simulink model "ADA"  (R2019b)
settings: Solver=FixedStepAuto  StartTime=0.0  StopTime=10.0  FixedStep=fixedStepSize  RelTol=1e-3
undefined symbols (not defined in the file): ADA_notAlwaysHorizon, ADA_subsystem1_rpmLimit, ADA_subsystem1_timeHorizon, ADA_subsystem2_gear1, ADA_subsystem2_gear2, ADA_subsystem2_impellerMax, ADA_subsystem2_impellerMin, ADA_subsystem2_maxValue, ADA_subsystem2_throttleMin, ADA_subsystem3_gear, ADA_subsystem3_gearSelectionState, ADA_subsystem3_speedMax, ADA_subsystem3_speedMin, fixedStepSize
libraries: simulink x1
settings Model: Creator=JEDDELAN  LastModifiedBy=alex
settings DataIOCC: SaveOutput=off  SaveTime=off  ReturnWorkspaceOutputs=off
settings DebuggingCC: ArithmeticOperatorsInVariantConditions=warning
settings SFSimCC: SimUseLocalCustomCode=off  CustomCodeUndefinedFunction=UseInterfaceOnly
settings RTWCC: RTWUseLocalCustomCode=off
settings GRTTargetCC: CombineOutputUpdateFcns=off  MatFileLogging=off

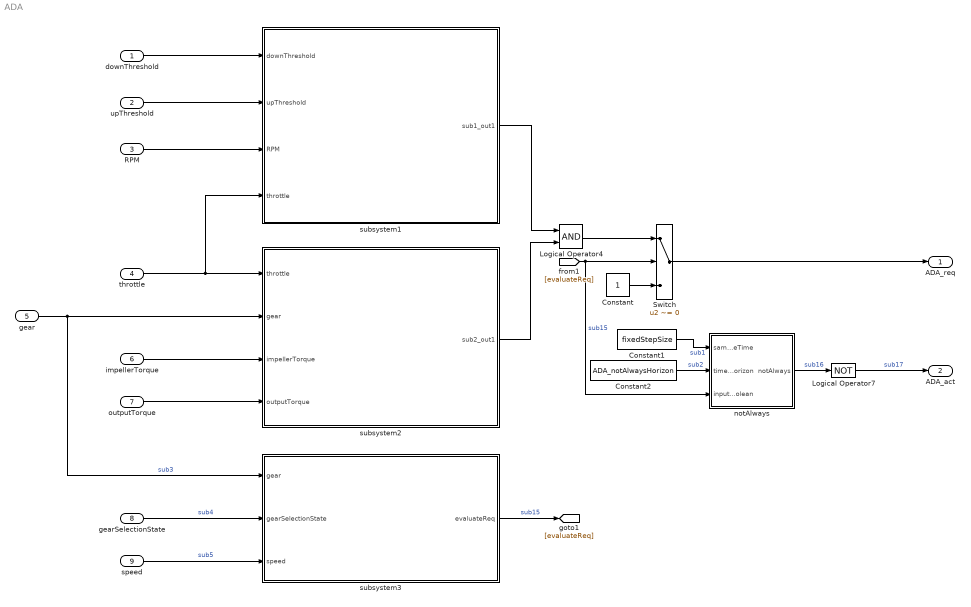
== system ADA ==
  downThreshold : Inport  OutDataTypeStr=double
  upThreshold : Inport  Port=2  OutDataTypeStr=double
  RPM : Inport  Description=|  Port=3  OutDataTypeStr=double  PortDimensions=1  BusOutputAsStruct=on
      | Engine Speed [rpm]
      | Engine Speed derivative [rpm/s]
  throttle : Inport  Port=4
  gear : Inport  Port=5
  impellerTorque : Inport  Port=6
  outputTorque : Inport  Port=7
  gearSelectionState : Inport  Port=8
  speed : Inport  Port=9
  Constant : Constant  OutDataTypeStr=boolean
  Constant1 : Constant  Value=fixedStepSize
  Constant2 : Constant  Value=ADA_notAlwaysHorizon
  Logical Operator4 : Logic  AllPortsSameDT=off  OutDataTypeStr=boolean
  Logical Operator7 : Logic  Operator=NOT  AllPortsSameDT=off  OutDataTypeStr=boolean
  Switch : Switch  Criteria=u2 ~= 0
  notAlways : Subsystem
      settings: CopyFcn=set_param(gcbh,'LinkStatus','none');
  subsystem1 : Subsystem
  subsystem2 : Subsystem
  subsystem3 : Subsystem
  ADA_req : Outport  OutDataTypeStr=boolean  PortDimensions=1  VectorParamsAs1DForOutWhenUnconnected=off
  ADA_act : Outport  Port=2  OutDataTypeStr=boolean  PortDimensions=1  VectorParamsAs1DForOutWhenUnconnected=off
  wires:
  notAlways/1(notAlways) -> Logical Operator7/1  "sub16"
  [evaluateReq] -> Switch/2, notAlways/3(inputBoolean)  "sub15"
  Logical Operator4/1 -> Switch/1
  speed/1 -> subsystem3/3(speed)  "sub5"
  upThreshold/1 -> subsystem1/2(upThreshold)
  Logical Operator7/1 -> ADA_act/1  "sub17"
  throttle/1 -> subsystem2/1(throttle), subsystem1/4(throttle)
  impellerTorque/1 -> subsystem2/3(impellerTorque)
  RPM/1 -> subsystem1/3(RPM)
  subsystem3/1(evaluateReq) -> [evaluateReq]  "sub15"
  outputTorque/1 -> subsystem2/4(outputTorque)
  gear/1 -> subsystem3/1(gear), subsystem2/2(gear)  "sub3"
  Constant1/1 -> notAlways/1(sampleTime)  "sub1"
  subsystem2/1(sub2_out1) -> Logical Operator4/2
  Constant/1 -> Switch/3
  Switch/1 -> ADA_req/1
  gearSelectionState/1 -> subsystem3/2(gearSelectionState)  "sub4"
  Constant2/1 -> notAlways/2(timeHorizon)  "sub2"
  downThreshold/1 -> subsystem1/1(downThreshold)
  subsystem1/1(sub1_out1) -> Logical Operator4/1

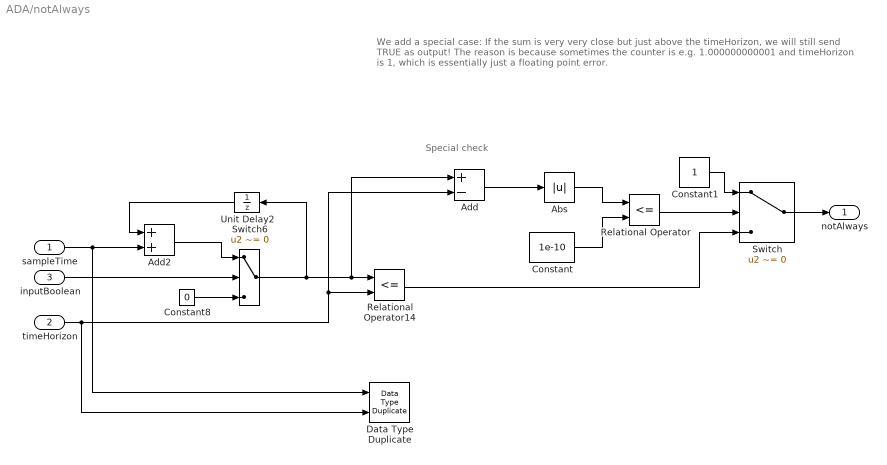
== system ADA/notAlways ==
  note: Special check
  note: We add a special case:
      | If the sum is very very close but just above the timeHorizon, we will still send TRUE as output!
      |
      | The reason is because sometimes the counter is e.g. 1.000000000001 and timeHorizon is 1, which is essentially just a floating point error.
  sampleTime : Inport
  timeHorizon : Inport  Port=2
  inputBoolean : Inport  Port=3
  Abs : Abs
  Add : Sum  Inputs=+-
  Add2 : Sum
  Constant : Constant  Value=1e-10
  Constant1 : Constant  OutDataTypeStr=boolean
  Constant8 : Constant  Value=0  OutDataTypeStr=Inherit: Inherit via back propagation
  Data Type Duplicate : DataTypeDuplicate
  Relational Operator : RelationalOperator  Operator=<=  OutDataTypeStr=boolean  RndMeth=Simplest
  Relational Operator14 : RelationalOperator  Operator=<=  OutDataTypeStr=boolean  RndMeth=Nearest
  Switch : Switch  Criteria=u2 ~= 0
  Switch6 : Switch  Criteria=u2 ~= 0
  Unit Delay2 : UnitDelay  SampleTime=-1  HasFrameUpgradeWarning=on
  notAlways : Outport  VectorParamsAs1DForOutWhenUnconnected=off
  wires:
  Switch6/1 -> Add/1, Relational Operator14/1, Unit Delay2/1
  timeHorizon/1 -> Add/2, Relational Operator14/2, Data Type Duplicate/2
  Relational Operator14/1 -> Switch/3
  Unit Delay2/1 -> Add2/1
  Add2/1 -> Switch6/1
  sampleTime/1 -> Add2/2, Data Type Duplicate/1
  Constant8/1 -> Switch6/3
  inputBoolean/1 -> Switch6/2
  Add/1 -> Abs/1
  Abs/1 -> Relational Operator/1
  Constant/1 -> Relational Operator/2
  Relational Operator/1 -> Switch/2
  Constant1/1 -> Switch/1
  Switch/1 -> notAlways/1

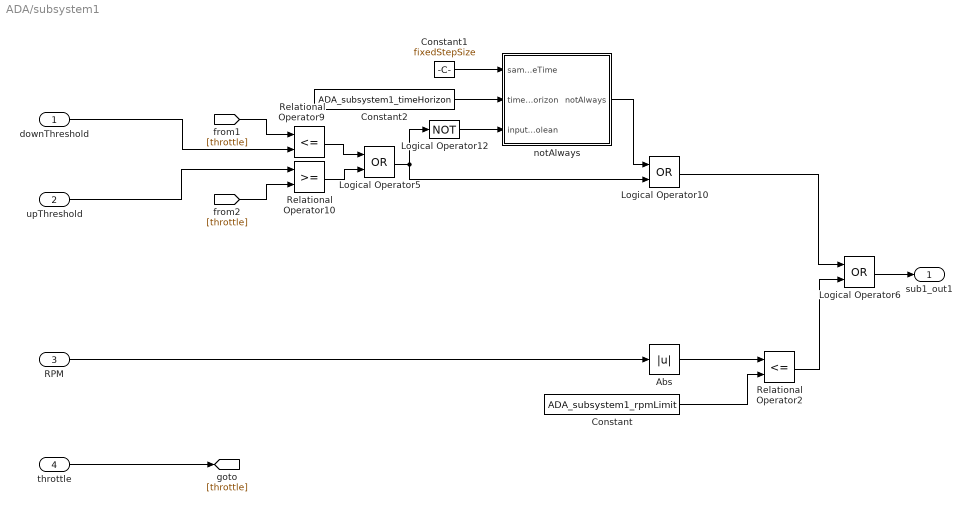
== system ADA/subsystem1 ==
  downThreshold : Inport
  upThreshold : Inport  Port=2
  RPM : Inport  Port=3
  throttle : Inport  Port=4
  Abs : Abs
  Constant : Constant  Value=ADA_subsystem1_rpmLimit
  Constant1 : Constant  Value=fixedStepSize
  Constant2 : Constant  Value=ADA_subsystem1_timeHorizon
  Logical Operator10 : Logic  Operator=OR  AllPortsSameDT=off  OutDataTypeStr=boolean
  Logical Operator12 : Logic  Operator=NOT  AllPortsSameDT=off  OutDataTypeStr=boolean
  Logical Operator5 : Logic  Operator=OR  AllPortsSameDT=off  OutDataTypeStr=boolean
  Logical Operator6 : Logic  Operator=OR  AllPortsSameDT=off  OutDataTypeStr=boolean
  Relational Operator10 : RelationalOperator  OutDataTypeStr=boolean  RndMeth=Nearest
  Relational Operator2 : RelationalOperator  Operator=<=  OutDataTypeStr=boolean  RndMeth=Nearest
  Relational Operator9 : RelationalOperator  Operator=<=  OutDataTypeStr=boolean  RndMeth=Nearest
  notAlways : Subsystem
      settings: CopyFcn=set_param(gcbh,'LinkStatus','none');
  sub1_out1 : Outport  VectorParamsAs1DForOutWhenUnconnected=off
  wires:
  throttle/1 -> [throttle]
  notAlways/1(notAlways) -> Logical Operator10/1
  Constant2/1 -> notAlways/2(timeHorizon)
  Constant1/1 -> notAlways/1(sampleTime)
  Logical Operator12/1 -> notAlways/3(inputBoolean)
  Logical Operator5/1 -> Logical Operator10/2, Logical Operator12/1
  Logical Operator10/1 -> Logical Operator6/1
  RPM/1 -> Abs/1
  Constant/1 -> Relational Operator2/2
  Abs/1 -> Relational Operator2/1
  Relational Operator2/1 -> Logical Operator6/2
  downThreshold/1 -> Relational Operator9/2
  [throttle] -> Relational Operator9/1
  Relational Operator9/1 -> Logical Operator5/1
  [throttle] -> Relational Operator10/2
  Relational Operator10/1 -> Logical Operator5/2
  Logical Operator6/1 -> sub1_out1/1
  upThreshold/1 -> Relational Operator10/1

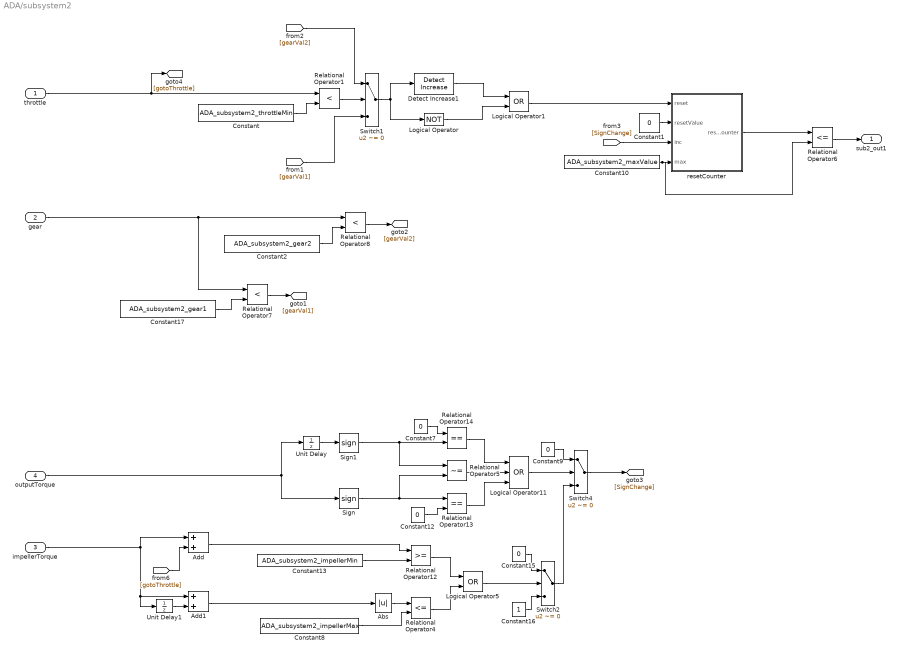
== system ADA/subsystem2 ==
  throttle : Inport
  gear : Inport  Port=2
  impellerTorque : Inport  Port=3
  outputTorque : Inport  Port=4
  Abs : Abs
  Add : Sum
  Add1 : Sum
  Constant : Constant  Value=ADA_subsystem2_throttleMin
  Constant{1,7,9,12,15} (5 alike) : Constant  Value=0
  Constant10 : Constant  Value=ADA_subsystem2_maxValue
  Constant13 : Constant  Value=ADA_subsystem2_impellerMin
  Constant16 : Constant
  Constant17 : Constant  Value=ADA_subsystem2_gear1
  Constant2 : Constant  Value=ADA_subsystem2_gear2
  Constant8 : Constant  Value=ADA_subsystem2_impellerMax
  Detect Increase1 : simulink/Logic and Bit Operations/Detect Increase  vinit=0.0  OutDataTypeStr=boolean
  Logical Operator : Logic  Operator=NOT  AllPortsSameDT=off  OutDataTypeStr=boolean
  Logical Operator1 : Logic  Operator=OR  AllPortsSameDT=off  OutDataTypeStr=boolean
  Logical Operator11 : Logic  Operator=OR  Inputs=3  AllPortsSameDT=off  OutDataTypeStr=boolean
  Logical Operator5 : Logic  Operator=OR  AllPortsSameDT=off  OutDataTypeStr=boolean
  Relational Operator1 : RelationalOperator  Operator=<  OutDataTypeStr=boolean  RndMeth=Nearest
  Relational Operator12 : RelationalOperator  OutDataTypeStr=boolean  RndMeth=Nearest
  Relational Operator13 : RelationalOperator  Operator===  OutDataTypeStr=boolean  RndMeth=Nearest
  Relational Operator14 : RelationalOperator  Operator===  OutDataTypeStr=boolean  RndMeth=Nearest
  Relational Operator4 : RelationalOperator  Operator=<=  OutDataTypeStr=boolean  RndMeth=Nearest
  Relational Operator5 : RelationalOperator  Operator=~=  OutDataTypeStr=boolean  RndMeth=Nearest
  Relational Operator6 : RelationalOperator  Operator=<=  OutDataTypeStr=boolean  RndMeth=Nearest
  Relational Operator7 : RelationalOperator  Operator=<  OutDataTypeStr=boolean  RndMeth=Nearest
  Relational Operator8 : RelationalOperator  Operator=<  OutDataTypeStr=boolean  RndMeth=Nearest
  Sign : Signum
  Sign1 : Signum
  Switch1 : Switch  Criteria=u2 ~= 0
  Switch2 : Switch  Criteria=u2 ~= 0
  Switch4 : Switch  Criteria=u2 ~= 0
  Unit Delay : UnitDelay  SampleTime=-1  HasFrameUpgradeWarning=on
  Unit Delay1 : UnitDelay  SampleTime=-1  HasFrameUpgradeWarning=on
  resetCounter : Subsystem
      settings: CopyFcn=set_param(gcbh,'LinkStatus','none');
  sub2_out1 : Outport  VectorParamsAs1DForOutWhenUnconnected=off
  wires:
  Logical Operator5/1 -> Switch2/2
  Relational Operator4/1 -> Logical Operator5/2
  Abs/1 -> Relational Operator4/1
  Constant8/1 -> Relational Operator4/2
  Add1/1 -> Abs/1
  Unit Delay1/1 -> Add1/2
  Constant7/1 -> Relational Operator14/1
  [SignChange] -> resetCounter/3(inc)
  Logical Operator1/1 -> resetCounter/1(reset)
  throttle/1 -> Relational Operator1/1, [gotoThrottle]
  [gearVal2] -> Switch1/1
  [gearVal1] -> Switch1/3
  Relational Operator1/1 -> Switch1/2
  Constant/1 -> Relational Operator1/2
  Constant15/1 -> Switch2/1
  Switch2/1 -> Switch4/3
  Relational Operator14/1 -> Logical Operator11/1
  Constant12/1 -> Relational Operator13/2
  Relational Operator13/1 -> Logical Operator11/3
  Relational Operator5/1 -> Logical Operator11/2
  Constant16/1 -> Switch2/3
  Logical Operator11/1 -> Switch4/2
  Relational Operator12/1 -> Logical Operator5/1
  Constant13/1 -> Relational Operator12/2
  Add/1 -> Relational Operator12/1
  impellerTorque/1 -> Add/1, Unit Delay1/1, Add1/1
  [gotoThrottle] -> Add/2
  gear/1 -> Relational Operator7/1, Relational Operator8/1
  outputTorque/1 -> Unit Delay/1, Sign/1
  Unit Delay/1 -> Sign1/1
  Sign1/1 -> Relational Operator5/1, Relational Operator14/2
  Sign/1 -> Relational Operator5/2, Relational Operator13/1
  Constant9/1 -> Switch4/1
  Switch4/1 -> [SignChange]
  resetCounter/1(resetCounter) -> Relational Operator6/1
  Constant1/1 -> resetCounter/2(resetValue)
  Constant10/1 -> Relational Operator6/2, resetCounter/4(max)
  Switch1/1 -> Detect Increase1/1, Logical Operator/1
  Detect Increase1/1 -> Logical Operator1/1
  Logical Operator/1 -> Logical Operator1/2
  Relational Operator6/1 -> sub2_out1/1
  Constant17/1 -> Relational Operator7/2
  Constant2/1 -> Relational Operator8/2
  Relational Operator7/1 -> [gearVal1]
  Relational Operator8/1 -> [gearVal2]

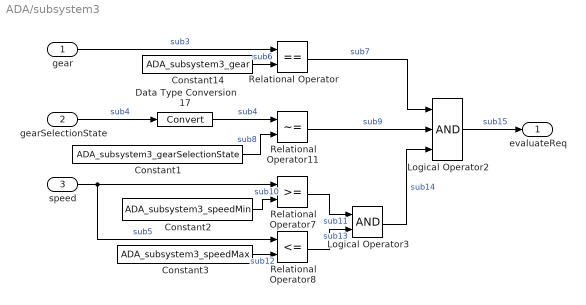
== system ADA/subsystem3 ==
  gear : Inport
  gearSelectionState : Inport  Port=2
  speed : Inport  Port=3
  Constant1 : Constant  Value=ADA_subsystem3_gearSelectionState
  Constant14 : Constant  Value=ADA_subsystem3_gear
  Constant2 : Constant  Value=ADA_subsystem3_speedMin
  Constant3 : Constant  Value=ADA_subsystem3_speedMax
  Data Type Conversion17 : DataTypeConversion
  Logical Operator2 : Logic  Inputs=3  AllPortsSameDT=off  OutDataTypeStr=boolean
  Logical Operator3 : Logic  AllPortsSameDT=off  OutDataTypeStr=boolean
  Relational Operator : RelationalOperator  Operator===  OutDataTypeStr=boolean  RndMeth=Nearest
  Relational Operator11 : RelationalOperator  Operator=~=  OutDataTypeStr=boolean  RndMeth=Nearest
  Relational Operator7 : RelationalOperator  OutDataTypeStr=boolean  RndMeth=Nearest
  Relational Operator8 : RelationalOperator  Operator=<=  OutDataTypeStr=boolean  RndMeth=Nearest
  evaluateReq : Outport  VectorParamsAs1DForOutWhenUnconnected=off
  wires:
  Relational Operator/1 -> Logical Operator2/1  "sub7"
  Relational Operator11/1 -> Logical Operator2/2  "sub9"
  Data Type Conversion17/1 -> Relational Operator11/1  "sub4"
  Constant1/1 -> Relational Operator11/2  "sub8"
  gearSelectionState/1 -> Data Type Conversion17/1  "sub4"
  Constant14/1 -> Relational Operator/2  "sub6"
  Logical Operator2/1 -> evaluateReq/1  "sub15"
  speed/1 -> Relational Operator8/1, Relational Operator7/1  "sub5"
  Constant2/1 -> Relational Operator7/2  "sub10"
  Relational Operator7/1 -> Logical Operator3/1  "sub11"
  Relational Operator8/1 -> Logical Operator3/2  "sub13"
  Constant3/1 -> Relational Operator8/2  "sub12"
  gear/1 -> Relational Operator/1  "sub3"
  Logical Operator3/1 -> Logical Operator2/3  "sub14"

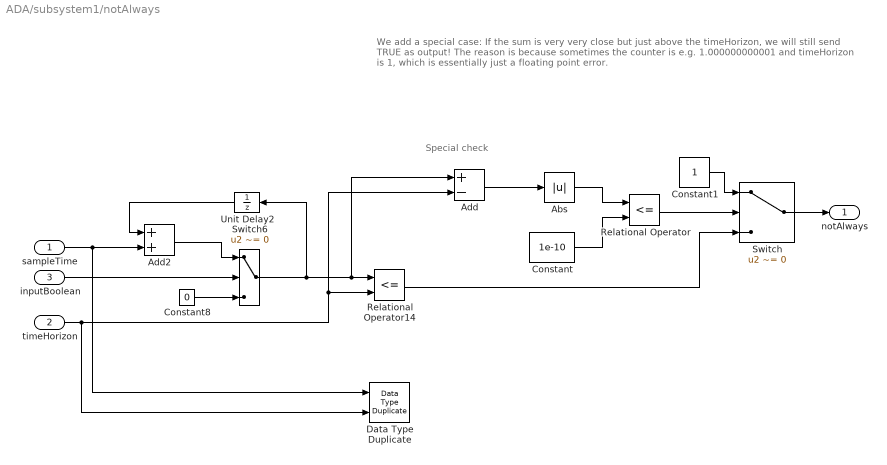
== system ADA/subsystem1/notAlways ==
  note: Special check
  note: We add a special case:
      | If the sum is very very close but just above the timeHorizon, we will still send TRUE as output!
      |
      | The reason is because sometimes the counter is e.g. 1.000000000001 and timeHorizon is 1, which is essentially just a floating point error.
  sampleTime : Inport
  timeHorizon : Inport  Port=2
  inputBoolean : Inport  Port=3
  Abs : Abs
  Add : Sum  Inputs=+-
  Add2 : Sum
  Constant : Constant  Value=1e-10
  Constant1 : Constant  OutDataTypeStr=boolean
  Constant8 : Constant  Value=0  OutDataTypeStr=Inherit: Inherit via back propagation
  Data Type Duplicate : DataTypeDuplicate
  Relational Operator : RelationalOperator  Operator=<=  OutDataTypeStr=boolean  RndMeth=Simplest
  Relational Operator14 : RelationalOperator  Operator=<=  OutDataTypeStr=boolean  RndMeth=Nearest
  Switch : Switch  Criteria=u2 ~= 0
  Switch6 : Switch  Criteria=u2 ~= 0
  Unit Delay2 : UnitDelay  SampleTime=-1  HasFrameUpgradeWarning=on
  notAlways : Outport  VectorParamsAs1DForOutWhenUnconnected=off
  wires:
  Switch6/1 -> Add/1, Relational Operator14/1, Unit Delay2/1
  timeHorizon/1 -> Add/2, Relational Operator14/2, Data Type Duplicate/2
  Relational Operator14/1 -> Switch/3
  Unit Delay2/1 -> Add2/1
  Add2/1 -> Switch6/1
  sampleTime/1 -> Add2/2, Data Type Duplicate/1
  Constant8/1 -> Switch6/3
  inputBoolean/1 -> Switch6/2
  Add/1 -> Abs/1
  Abs/1 -> Relational Operator/1
  Constant/1 -> Relational Operator/2
  Relational Operator/1 -> Switch/2
  Constant1/1 -> Switch/1
  Switch/1 -> notAlways/1

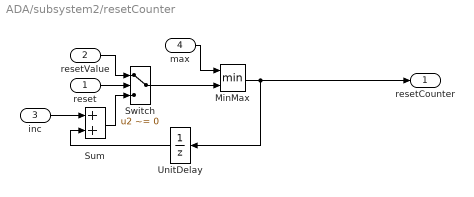
== system ADA/subsystem2/resetCounter ==
  reset : Inport
  resetValue : Inport  Port=2
  inc : Inport  Port=3
  max : Inport  Port=4
  MinMax : MinMax  Tag=struct('comment',struct('text','','placement',1),'inputs','2','logdata',struct('maxnumvals',4096,'plotchannels',[],'loggingmode',3,'channels',1),'output',struct('width',1,'name','$S_$B','unit','','type','Float32','offset',0,'max',NaN,'min',NaN,'freeze',1,'lsb',1,'arb',0,'class','default','address','','description','','autoscalingmode',1,'lowerheadroom',1,'upperheadroom',1,'headroomunit','bit','checkmin',0,'checkmax',0,'show',0,'variable','','scaling','','keepdatatype',1,'castoutput',0),'function','min','date',734124.44480996532,'scalingvalid',0)  Inputs=2  OutDataTypeStr=Inherit: Inherit via back propagation  InputSameDT=on
  Sum : Sum  Tag=struct('comment',struct('text','','placement',1),'logdata',struct('maxnumvals',4096,'plotchannels',[],'loggingmode',3,'channels',1),'output',struct('width',1,'name','$S_$B','unit','','type','Float32','offset',0,'max',NaN,'min',NaN,'freeze',1,'lsb',1,'arb',0,'class','default','address','','description','','autoscalingmode',1,'lowerheadroom',1,'upperheadroom',1,'headroomunit','bit','checkmin',0,'checkmax',0,'show',0,'variable','','scaling','','keepdatatype',1,'castoutput',0),'inputs','++','date',734124.44480996532,'scalingvalid',0)  OutDataTypeStr=Inherit: Same as accumulator  InputSameDT=on
  Switch : Switch  Tag=struct('comment',struct('text','','placement',1),'logdata',struct('maxnumvals',4096,'plotchannels',[],'loggingmode',3,'channels',1),'output',struct('width',1,'name','$S_$B','unit','','type','Float32','offset',0,'max',NaN,'min',NaN,'freeze',1,'lsb',1,'arb',0,'class','default','address','','description','','autoscalingmode',1,'lowerheadroom',1,'upperheadroom',1,'headroomunit','bit','checkmin',0,'checkmax',0,'show',0,'variable','','scaling','','keepdatatype',1,'castoutput',0),'threshold',struct('width',1,'name','$S_$B_threshold','unit','','type','Int16','offset',0,'max',NaN,'min',NaN,'freeze',1,'lsb',1,'arb',0,'class','default','address','','description','','value','0.5','scalar',0,'variable','','scaling','','keepdatatype',1,'criteria',1),'date',734124.4448101389,'scalingvalid',0)  Criteria=u2 ~= 0  Threshold=0.5  InputSameDT=on
  UnitDelay : UnitDelay  Tag=struct('comment',struct('text','','placement',1),'logdata',struct('maxnumvals',4096,'plotchannels',[],'loggingmode',3,'channels',1),'output',struct('width',1,'name','$S_$B','unit','','type','Float32','offset',0,'max',NaN,'min',NaN,'freeze',1,'lsb',1,'arb',0,'class','default','address','','description','','autoscalingmode',1,'lowerheadroom',1,'upperheadroom',1,'headroomunit','bit','checkmin',0,'checkmax',0,'show',0,'variable','','scaling','','keepdatatype',1,'castoutput',0),'state',struct('variable','','description','','name','X_$S_$B','width',1,'address','','max',NaN,'min',NaN,'class','default','type','Float32','scaling','','lsb',1,'offset',0,'arb',0,'freeze',1,'unit','','initial','0'),'dt','-1','date',734124.44481032412,'scalingvalid',0)  SampleTime=-1  HasFrameUpgradeWarning=on
  resetCounter : Outport  VectorParamsAs1DForOutWhenUnconnected=off
  wires:
  UnitDelay/1 -> Sum/2
  max/1 -> MinMax/1
  Switch/1 -> MinMax/2
  MinMax/1 -> UnitDelay/1, resetCounter/1
  Sum/1 -> Switch/3
  resetValue/1 -> Switch/1
  inc/1 -> Sum/1
  reset/1 -> Switch/2
